simulink model "DFIItvertical"  (R2016a)
settings: Solver=VariableStepAuto  StartTime=0.0  StopTime=10.0  RelTol=1e-3
undefined symbols (not defined in the file or in its folder): a1, a2, a3, b0, b1, b2, b3
settings Model: Creator=thib  LastModifiedBy=thib

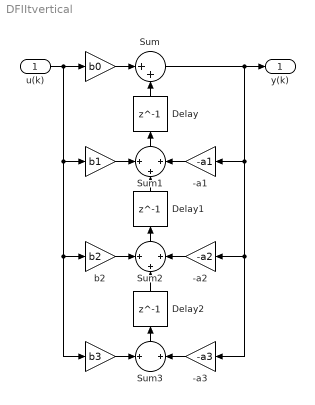
== system DFIItvertical ==
  "u(k) " : Inport
  " " : Gain  Gain=b0
  " " : Gain  Gain=b1
  " " : Gain  Gain=b3
  -a1 : Gain  Gain=-a1
  -a2 : Gain  Gain=-a2
  -a3 : Gain  Gain=-a3
  Delay : Delay  DelayLength=1  InitialCondition=0
  Delay1 : Delay  DelayLength=1  InitialCondition=0
  Delay2 : Delay  DelayLength=1  InitialCondition=0
  Sum : Sum  Inputs=|++
  Sum1 : Sum  Inputs=+|+|+
  Sum2 : Sum  Inputs=+|+|+
  Sum3 : Sum  Inputs=+||+
  b2 : Gain  Gain=b2
  y(k) : Outport
  wires:
  " "/1 -> Sum/1
  Delay/1 -> Sum/2
  " "/1 -> Sum1/1
  Sum1/1 -> Delay/1
  -a1/1 -> Sum1/3
  b2/1 -> Sum2/1
  -a2/1 -> Sum2/3
  Delay1/1 -> Sum1/2
  Sum2/1 -> Delay1/1
  "u(k) "/1 -> " "/1, b2/1, " "/1, " "/1
  " "/1 -> Sum3/1
  Sum/1 -> -a3/1, -a2/1, -a1/1, y(k)/1
  Sum3/1 -> Delay2/1
  Delay2/1 -> Sum2/2
  -a3/1 -> Sum3/2
